simulink model "SPWMinverter3P_Final"  (Simulink 10.0)
settings: Solver=ode3  StartTime=0.0  StopTime=0.04  RelTol=1e-3  EnableMultiTasking=on
libraries: powerlib x16
settings Model: Creator=Administrator  LastModifiedBy=bhisma
settings SolverCC: PositivePriorityOrder=on
settings DataIOCC: LimitDataPoints=on  SignalLoggingSaveFormat=ModelDataLogs
settings OptimizationCC: ExpressionDepthLimit=2147483647
settings DebuggingCC: SolverPrmCheckMsg=warning  FcnCallInpInsideContextMsg=warning  StateNameClashWarn=warning
settings SFSimCC: SimParseCustomCode=off
settings GRTTargetCC: GeneratePreprocessorConditionals=Disable all
settings ConfigComp: CovExternalEMLEnable=off
settings SimscapeCC: SimscapeNormalizeSystem=off

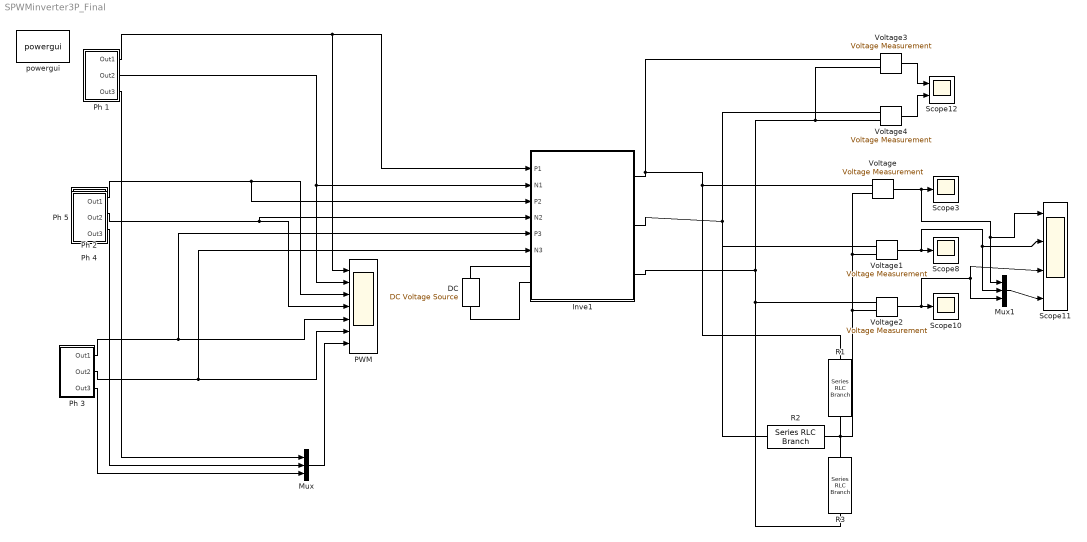
== system SPWMinverter3P_Final ==
  DC : powerlib/Electrical Sources/DC Voltage Source  SystemSampleTime=-1  Amplitude=10  Measurements=None
      settings: SourceProductName=Simscape Electrical
  Inve1 : Subsystem
  Mux : Mux  Inputs=3
  Mux1 : Mux  Inputs=3
  PWM : Scope  NumInputPorts=7
  Ph 1 : Subsystem  mask{SA=3, CA=3, Sf=50, Cf=5000}
      mask prompts: SA "Sine Amplitude"; CA "Carrier Amplitude"; Sf "Sine Frequency"; Cf "Carrier Frequency"
  Ph 2 : Subsystem  mask{SA=3, CA=3, Sf=50, Cf=5000}
      mask prompts: SA "Sine Amplitude"; CA "Carrier Amplitude"; Sf "Sine Frequency"; Cf "Carrier Frequency"
  Ph 3 : Subsystem  mask{SA=3, CA=3, Sf=50, Cf=5000}
      mask prompts: SA "Sine Amplitude"; CA "Carrier Amplitude"; Sf "Sine Frequency"; Cf "Carrier Frequency"
  Ph 4 : Subsystem  mask{SA=3, CA=3, Sf=50, Cf=5000}
      mask prompts: SA "Sine Amplitude"; CA "Carrier Amplitude"; Sf "Sine Frequency"; Cf "Carrier Frequency"
  Ph 5 : Subsystem  mask{SA=3, CA=3, Sf=50, Cf=5000}
      mask prompts: SA "Sine Amplitude"; CA "Carrier Amplitude"; Sf "Sine Frequency"; Cf "Carrier Frequency"
  R1 : powerlib/Elements/Series RLC Branch  PhysicalDomain=powersysdomain  SubClassName=unknown  LeftPortType=p1  RightPortType=p1  LConnTagsString=__new0  RConnTagsString=__new0  BranchType=R  Resistance=10  Inductance=1e-3  SetiL0=off  InitialCurrent=0  Capacitance=1e-6  Setx0=off  InitialVoltage=0  Measurements=None
      settings: SourceProductName=Simscape Electrical
  R2 : powerlib/Elements/Series RLC Branch  PhysicalDomain=powersysdomain  SubClassName=unknown  LeftPortType=p1  RightPortType=p1  LConnTagsString=__new0  RConnTagsString=__new0  BranchType=R  Resistance=10  Inductance=1e-3  SetiL0=off  InitialCurrent=0  Capacitance=1e-6  Setx0=off  InitialVoltage=0  Measurements=None
      settings: SourceProductName=Simscape Electrical
  R3 : powerlib/Elements/Series RLC Branch  PhysicalDomain=powersysdomain  SubClassName=unknown  LeftPortType=p1  RightPortType=p1  LConnTagsString=__new0  RConnTagsString=__new0  BranchType=R  Resistance=10  Inductance=1e-3  SetiL0=off  InitialCurrent=0  Capacitance=1e-6  Setx0=off  InitialVoltage=0  Measurements=None
      settings: SourceProductName=Simscape Electrical
  Scope10 : Scope
  Scope11 : Scope  NumInputPorts=4
  Scope12 : Scope  NumInputPorts=2
  Scope3 : Scope
  Scope8 : Scope
  Voltage{,1..4} (5 alike) : powerlib/Measurements/Voltage Measurement  SystemSampleTime=-1  PhasorSimulation=off  OutputType=Complex  PSBequivalent=0
      settings: SourceProductName=Simscape Electrical
  powergui : powerlib/powergui  Priority=1  SystemSampleTime=-1  SimulationMode=Continuous  SampleTime=50e-6  frequency=60  SPID=off  DisableSnubberDevices=off  DisableRonSwitches=off  DisableVfSwitches=off  SwTol=0  Interpol=off  frequencyindice=0  echomessages=off  HookPort=off  DisplayEquations=off  FunctionMessages=off  EnableUseOfTLC=off  x0status=blocks  RestoreLinks=warning  ResistiveCurrentMeasurement=off  Ylog=off  Xlog=on  ShowGrid=off  save=off  variable=ZData  ZoomFFT=off  StartTime=0.0  cycles=1  DisplayStyle=1  FreqAxis=off  MaxFrequency=1000  frequencyindicesteady=1  display=off  methode=off
      settings: SourceProductName=Simscape Electrical
  wires:
  Voltage/1 -> Scope11/1, Mux1/1, Scope3/1
  Mux/1 -> PWM/7
  Voltage1/1 -> Scope8/1, Scope11/2, Mux1/2
  Voltage2/1 -> Scope10/1, Scope11/3, Mux1/3
  Mux1/1 -> Scope11/4
  Voltage3/1 -> Scope12/1
  Voltage4/1 -> Scope12/2
  Ph 1/1(Out1) -> Inve1/1(P1), PWM/1
  Ph 1/2(Out2) -> Inve1/2(N1), PWM/2
  Ph 1/3(Out3) -> Mux/1
  Ph 2/1(Out1) -> Inve1/3(P2), PWM/3
  Ph 2/2(Out2) -> Inve1/4(N2), PWM/4
  Ph 2/3(Out3) -> Mux/2
  Ph 3/1(Out1) -> Inve1/5(P3), PWM/5
  Ph 3/2(Out2) -> Inve1/6(N3), PWM/6
  Ph 3/3(Out3) -> Mux/3
  connections:
  DC/RConn1 -- Inve1/LConn1
  Inve1/LConn2 -- DC/LConn1
  R1/RConn1 -- Voltage2/LConn2 -- Voltage1/LConn2 -- Voltage/LConn2 -- R3/RConn1 -- R2/LConn1
  R2/RConn1 -- Inve1/RConn2 -- Voltage4/LConn1 -- Voltage1/LConn1
  R3/LConn1 -- Voltage2/LConn1 -- Inve1/RConn3 -- Voltage4/LConn2 -- Voltage3/LConn2
  Inve1/RConn1 -- Voltage3/LConn1 -- R1/LConn1 -- Voltage/LConn1

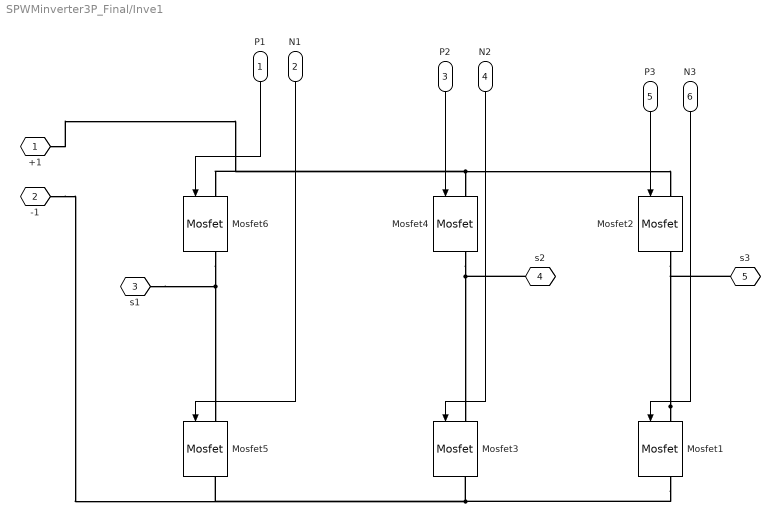
== system SPWMinverter3P_Final/Inve1 ==
  P1 : Inport
  N1 : Inport  Port=2
  P2 : Inport  Port=3
  N2 : Inport  Port=4
  P3 : Inport  Port=5
  N3 : Inport  Port=6
  Mosfet{1..6} (6 alike) : powerlib/Power Electronics/Mosfet  SystemSampleTime=-1  Ron=0.1  Lon=0  Rd=0.01  Vfd=0  IC=0  Rs=1e5  Cs=inf  Measurements=on
      settings: SourceProductName=Simscape Electrical
  +1 : PMIOPort  Tag=PMCPort  Side=Left
  -1 : PMIOPort  Tag=PMCPort  Port=2  Side=Left
  s1 : PMIOPort  Tag=PMCPort  Port=3  Side=Right
  s2 : PMIOPort  Tag=PMCPort  Port=4  Side=Right
  s3 : PMIOPort  Tag=PMCPort  Port=5  Side=Right
  wires:
  P1/1 -> Mosfet6/1
  N1/1 -> Mosfet5/1
  P2/1 -> Mosfet4/1
  N2/1 -> Mosfet3/1
  P3/1 -> Mosfet2/1
  N3/1 -> Mosfet1/1
  connections:
  Mosfet5/RConn1 -- -1/RConn1 -- Mosfet3/RConn1 -- Mosfet1/RConn1
  Mosfet6/LConn1 -- +1/RConn1 -- Mosfet4/LConn1 -- Mosfet2/LConn1
  Mosfet6/RConn1 -- Mosfet5/LConn1 -- s1/RConn1
  s2/RConn1 -- Mosfet4/RConn1 -- Mosfet3/LConn1
  Mosfet1/LConn1 -- s3/RConn1 -- Mosfet2/RConn1

== system SPWMinverter3P_Final/Ph 1 ==
  PWM1 : Subsystem  mask{Deg=0}
      mask prompts: Deg "Degree"
  Scope : Scope  NumInputPorts=3
  Scope1 : Scope  NumInputPorts=4
  Out1 : Outport
  Out2 : Outport  Port=2
  Out3 : Outport  Port=3
  wires:
  PWM1/6(Out6) -> Scope1/3
  PWM1/5(Out5) -> Scope1/2, Out2/1
  PWM1/4(Out4) -> Scope1/1, Out1/1
  PWM1/3(Out3) -> Scope/3
  PWM1/2(Out2) -> Scope/2
  PWM1/1(Out1) -> Scope/1
  PWM1/7(Out7) -> Scope1/4, Out3/1

== system SPWMinverter3P_Final/Ph 2 ==
  PWM 2 : Subsystem  mask{Deg=120}
      mask prompts: Deg "Degree"
  Scope2 : Scope  NumInputPorts=3
  Scope4 : Scope  NumInputPorts=4
  Out1 : Outport
  Out2 : Outport  Port=2
  Out3 : Outport  Port=3
  wires:
  PWM 2/6(Out6) -> Scope4/3
  PWM 2/5(Out5) -> Scope4/2, Out2/1
  PWM 2/4(Out4) -> Scope4/1, Out1/1
  PWM 2/3(Out3) -> Scope2/3
  PWM 2/2(Out2) -> Scope2/2
  PWM 2/1(Out1) -> Scope2/1
  PWM 2/7(Out7) -> Scope4/4, Out3/1

== system SPWMinverter3P_Final/Ph 3 ==
  PWM 3 : Subsystem  mask{Deg=240}
      mask prompts: Deg "Degree"
  Scope5 : Scope  NumInputPorts=3
  Scope6 : Scope  NumInputPorts=4
  Out1 : Outport
  Out2 : Outport  Port=2
  Out3 : Outport  Port=3
  wires:
  PWM 3/6(Out6) -> Scope6/3
  PWM 3/5(Out5) -> Scope6/2, Out2/1
  PWM 3/4(Out4) -> Scope6/1, Out1/1
  PWM 3/3(Out3) -> Scope5/3
  PWM 3/2(Out2) -> Scope5/2
  PWM 3/1(Out1) -> Scope5/1
  PWM 3/7(Out7) -> Scope6/4, Out3/1

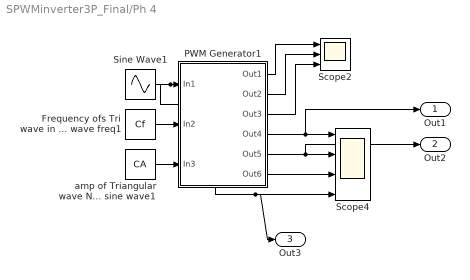
== system SPWMinverter3P_Final/Ph 4 ==
  Frequency ofs Tri wave in HZ note:It should < 2 times the sine wave freq1 : Constant  Value=Cf
  PWM Generator1 : Subsystem
  Scope2 : Scope  NumInputPorts=3
  Scope4 : Scope  NumInputPorts=4
  Sine Wave1 : Sin  Amplitude=SA  Frequency=2*pi*Sf  Phase=240*(pi/180)  SampleTime=0
  amp of Triangular wave Note:preferably the value of amp f sine wave1 : Constant  Value=CA
  Out1 : Outport
  Out2 : Outport  Port=2
  Out3 : Outport  Port=3
  wires:
  Sine Wave1/1 -> Out3/1, Scope4/4, PWM Generator1/1(In1)
  Frequency ofs Tri wave in HZ note:It should < 2 times the sine wave freq1/1 -> PWM Generator1/2(In2)
  amp of Triangular wave Note:preferably the value of amp f sine wave1/1 -> PWM Generator1/3(In3)
  PWM Generator1/1(Out1) -> Scope2/1
  PWM Generator1/2(Out2) -> Scope2/2
  PWM Generator1/3(Out3) -> Scope2/3
  PWM Generator1/4(Out4) -> Out1/1, Scope4/1
  PWM Generator1/5(Out5) -> Out2/1, Scope4/2
  PWM Generator1/6(Out6) -> Scope4/3

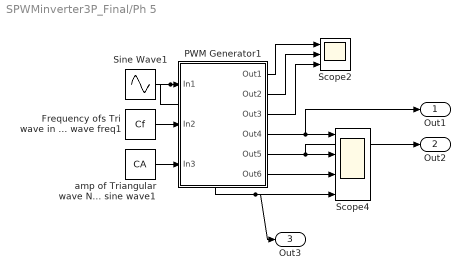
== system SPWMinverter3P_Final/Ph 5 ==
  Frequency ofs Tri wave in HZ note:It should < 2 times the sine wave freq1 : Constant  Value=Cf
  PWM Generator1 : Subsystem
  Scope2 : Scope  NumInputPorts=3
  Scope4 : Scope  NumInputPorts=4
  Sine Wave1 : Sin  Amplitude=SA  Frequency=2*pi*Sf  Phase=120*(pi/180)  SampleTime=0
  amp of Triangular wave Note:preferably the value of amp f sine wave1 : Constant  Value=CA
  Out1 : Outport
  Out2 : Outport  Port=2
  Out3 : Outport  Port=3
  wires:
  Sine Wave1/1 -> Out3/1, Scope4/4, PWM Generator1/1(In1)
  Frequency ofs Tri wave in HZ note:It should < 2 times the sine wave freq1/1 -> PWM Generator1/2(In2)
  amp of Triangular wave Note:preferably the value of amp f sine wave1/1 -> PWM Generator1/3(In3)
  PWM Generator1/1(Out1) -> Scope2/1
  PWM Generator1/2(Out2) -> Scope2/2
  PWM Generator1/3(Out3) -> Scope2/3
  PWM Generator1/4(Out4) -> Out1/1, Scope4/1
  PWM Generator1/5(Out5) -> Out2/1, Scope4/2
  PWM Generator1/6(Out6) -> Scope4/3

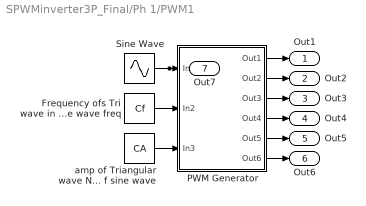
== system SPWMinverter3P_Final/Ph 1/PWM1 ==
  Frequency ofs Tri wave in HZ note:It should < 2 times the sine wave freq : Constant  Value=Cf
  PWM Generator : Subsystem
  Sine Wave : Sin  Amplitude=SA  Frequency=2*pi*Sf  Phase=Deg  SampleTime=0
  amp of Triangular wave Note:preferably the value of amp f sine wave : Constant  Value=CA
  Out1 : Outport
  Out2 : Outport  Port=2
  Out3 : Outport  Port=3
  Out4 : Outport  Port=4
  Out5 : Outport  Port=5
  Out6 : Outport  Port=6
  Out7 : Outport  Port=7
  wires:
  amp of Triangular wave Note:preferably the value of amp f sine wave/1 -> PWM Generator/3(In3)
  Frequency ofs Tri wave in HZ note:It should < 2 times the sine wave freq/1 -> PWM Generator/2(In2)
  Sine Wave/1 -> PWM Generator/1(In1), Out7/1
  PWM Generator/1(Out1) -> Out1/1
  PWM Generator/2(Out2) -> Out2/1
  PWM Generator/3(Out3) -> Out3/1
  PWM Generator/4(Out4) -> Out4/1
  PWM Generator/5(Out5) -> Out5/1
  PWM Generator/6(Out6) -> Out6/1

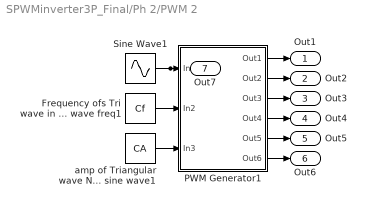
== system SPWMinverter3P_Final/Ph 2/PWM 2 ==
  Frequency ofs Tri wave in HZ note:It should < 2 times the sine wave freq1 : Constant  Value=Cf
  PWM Generator1 : Subsystem
  Sine Wave1 : Sin  Amplitude=SA  Frequency=2*pi*Sf  Phase=Deg*(pi/180)  SampleTime=0
  amp of Triangular wave Note:preferably the value of amp f sine wave1 : Constant  Value=CA
  Out1 : Outport
  Out2 : Outport  Port=2
  Out3 : Outport  Port=3
  Out4 : Outport  Port=4
  Out5 : Outport  Port=5
  Out6 : Outport  Port=6
  Out7 : Outport  Port=7
  wires:
  amp of Triangular wave Note:preferably the value of amp f sine wave1/1 -> PWM Generator1/3(In3)
  Frequency ofs Tri wave in HZ note:It should < 2 times the sine wave freq1/1 -> PWM Generator1/2(In2)
  Sine Wave1/1 -> PWM Generator1/1(In1), Out7/1
  PWM Generator1/1(Out1) -> Out1/1
  PWM Generator1/2(Out2) -> Out2/1
  PWM Generator1/3(Out3) -> Out3/1
  PWM Generator1/4(Out4) -> Out4/1
  PWM Generator1/5(Out5) -> Out5/1
  PWM Generator1/6(Out6) -> Out6/1

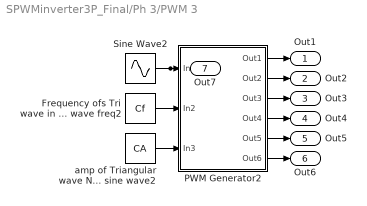
== system SPWMinverter3P_Final/Ph 3/PWM 3 ==
  Frequency ofs Tri wave in HZ note:It should < 2 times the sine wave freq2 : Constant  Value=Cf
  PWM Generator2 : Subsystem
  Sine Wave2 : Sin  Amplitude=SA  Frequency=2*pi*Sf  Phase=Deg*(pi/180)  SampleTime=0
  amp of Triangular wave Note:preferably the value of amp f sine wave2 : Constant  Value=CA
  Out1 : Outport
  Out2 : Outport  Port=2
  Out3 : Outport  Port=3
  Out4 : Outport  Port=4
  Out5 : Outport  Port=5
  Out6 : Outport  Port=6
  Out7 : Outport  Port=7
  wires:
  amp of Triangular wave Note:preferably the value of amp f sine wave2/1 -> PWM Generator2/3(In3)
  Frequency ofs Tri wave in HZ note:It should < 2 times the sine wave freq2/1 -> PWM Generator2/2(In2)
  Sine Wave2/1 -> PWM Generator2/1(In1), Out7/1
  PWM Generator2/1(Out1) -> Out1/1
  PWM Generator2/2(Out2) -> Out2/1
  PWM Generator2/3(Out3) -> Out3/1
  PWM Generator2/4(Out4) -> Out4/1
  PWM Generator2/5(Out5) -> Out5/1
  PWM Generator2/6(Out6) -> Out6/1

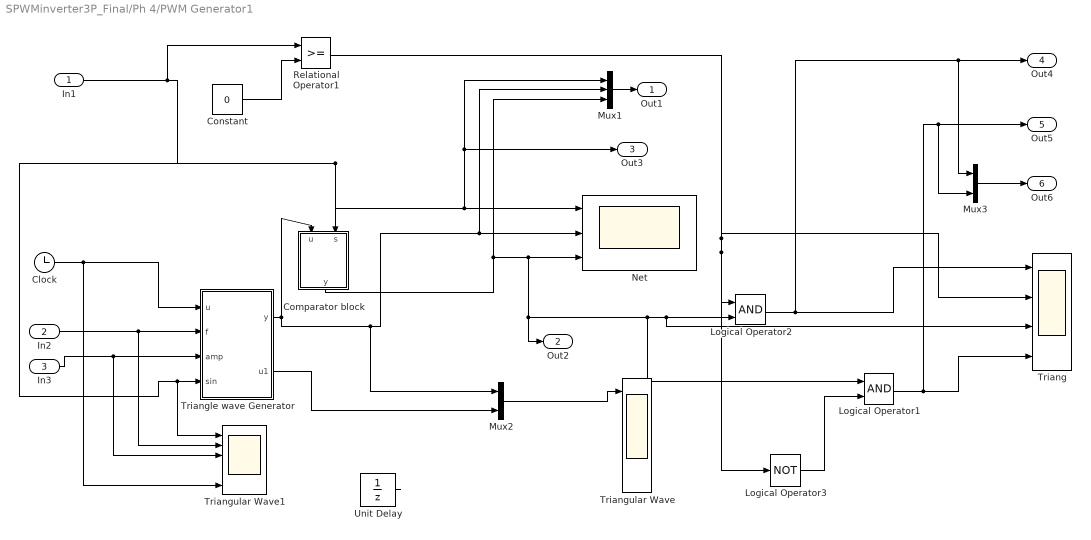
== system SPWMinverter3P_Final/Ph 4/PWM Generator1 ==
  In1 : Inport
  In2 : Inport  Port=2
  In3 : Inport  Port=3
  Clock : Clock
  Comparator block : MATLAB Function  TreatAsAtomicUnit=on
  Constant : Constant  Value=0
  Logical Operator1 : Logic  AllPortsSameDT=off  OutDataTypeStr=boolean
  Logical Operator2 : Logic  AllPortsSameDT=off  OutDataTypeStr=boolean
  Logical Operator3 : Logic  Operator=NOT  AllPortsSameDT=off  OutDataTypeStr=boolean
  Mux1 : Mux  Inputs=3
  Mux2 : Mux  Inputs=2
  Mux3 : Mux  Inputs=2
  Net : Scope  NumInputPorts=3
  Relational Operator1 : RelationalOperator  RndMeth=Nearest  InputSameDT=on
  Triang : Scope  NumInputPorts=4
  Triangle wave Generator : MATLAB Function  TreatAsAtomicUnit=on
  Triangular Wave : Scope  NumInputPorts=4
  Triangular Wave1 : Scope  NumInputPorts=6
  Unit Delay : UnitDelay  SampleTime=.01/10000
  Out1 : Outport
  Out2 : Outport  Port=2
  Out3 : Outport  Port=3
  Out4 : Outport  Port=4
  Out5 : Outport  Port=5
  Out6 : Outport  Port=6
  wires:
  Mux3/1 -> Out6/1
  Logical Operator1/1 -> Mux3/2, Out5/1, Triang/4
  Logical Operator3/1 -> Logical Operator1/2
  Logical Operator2/1 -> Mux3/1, Out4/1, Triang/1
  Relational Operator1/1 -> Logical Operator3/1, Logical Operator2/1, Triang/2
  Constant/1 -> Relational Operator1/2
  In3/1 -> Triangular Wave1/3, Triangle wave Generator/3(amp)
  In2/1 -> Triangular Wave1/2, Triangle wave Generator/2(f)
  Mux1/1 -> Out1/1
  Mux2/1 -> Triangular Wave/1
  Triangle wave Generator/2(u1) -> Mux2/2
  Comparator block/1(y) -> Logical Operator1/1, Triang/3, Logical Operator2/2, Out2/1, Net/3, Mux1/3
  In1/1 -> Relational Operator1/1, Triangular Wave1/1, Triangle wave Generator/4(sin), Comparator block/2(s), Net/1, Out3/1, Mux1/1
  Unit Delay/1 -> Unit Delay/1
  Triangle wave Generator/1(y) -> Mux2/1, Net/2, Mux1/2, Comparator block/1(u)
  Clock/1 -> Triangular Wave1/6, Triangle wave Generator/1(u)

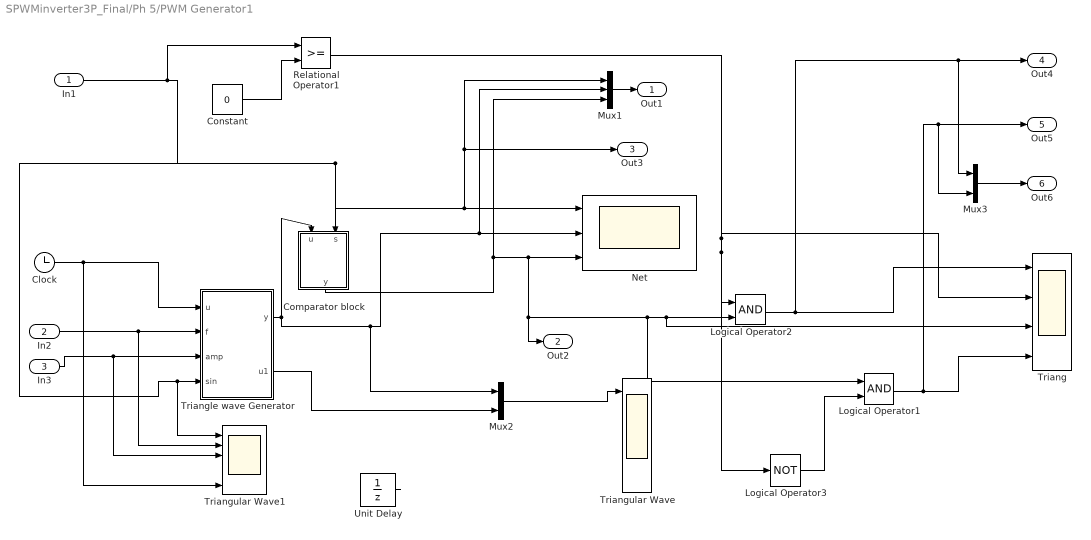
== system SPWMinverter3P_Final/Ph 5/PWM Generator1 ==
  In1 : Inport
  In2 : Inport  Port=2
  In3 : Inport  Port=3
  Clock : Clock
  Comparator block : MATLAB Function  TreatAsAtomicUnit=on
  Constant : Constant  Value=0
  Logical Operator1 : Logic  AllPortsSameDT=off  OutDataTypeStr=boolean
  Logical Operator2 : Logic  AllPortsSameDT=off  OutDataTypeStr=boolean
  Logical Operator3 : Logic  Operator=NOT  AllPortsSameDT=off  OutDataTypeStr=boolean
  Mux1 : Mux  Inputs=3
  Mux2 : Mux  Inputs=2
  Mux3 : Mux  Inputs=2
  Net : Scope  NumInputPorts=3
  Relational Operator1 : RelationalOperator  RndMeth=Nearest  InputSameDT=on
  Triang : Scope  NumInputPorts=4
  Triangle wave Generator : MATLAB Function  TreatAsAtomicUnit=on
  Triangular Wave : Scope  NumInputPorts=4
  Triangular Wave1 : Scope  NumInputPorts=6
  Unit Delay : UnitDelay  SampleTime=.01/10000
  Out1 : Outport
  Out2 : Outport  Port=2
  Out3 : Outport  Port=3
  Out4 : Outport  Port=4
  Out5 : Outport  Port=5
  Out6 : Outport  Port=6
  wires:
  Mux3/1 -> Out6/1
  Logical Operator1/1 -> Mux3/2, Out5/1, Triang/4
  Logical Operator3/1 -> Logical Operator1/2
  Logical Operator2/1 -> Mux3/1, Out4/1, Triang/1
  Relational Operator1/1 -> Logical Operator3/1, Logical Operator2/1, Triang/2
  Constant/1 -> Relational Operator1/2
  In3/1 -> Triangular Wave1/3, Triangle wave Generator/3(amp)
  In2/1 -> Triangular Wave1/2, Triangle wave Generator/2(f)
  Mux1/1 -> Out1/1
  Mux2/1 -> Triangular Wave/1
  Triangle wave Generator/2(u1) -> Mux2/2
  Comparator block/1(y) -> Logical Operator1/1, Triang/3, Logical Operator2/2, Out2/1, Net/3, Mux1/3
  In1/1 -> Relational Operator1/1, Triangular Wave1/1, Triangle wave Generator/4(sin), Comparator block/2(s), Net/1, Out3/1, Mux1/1
  Unit Delay/1 -> Unit Delay/1
  Triangle wave Generator/1(y) -> Mux2/1, Net/2, Mux1/2, Comparator block/1(u)
  Clock/1 -> Triangular Wave1/6, Triangle wave Generator/1(u)

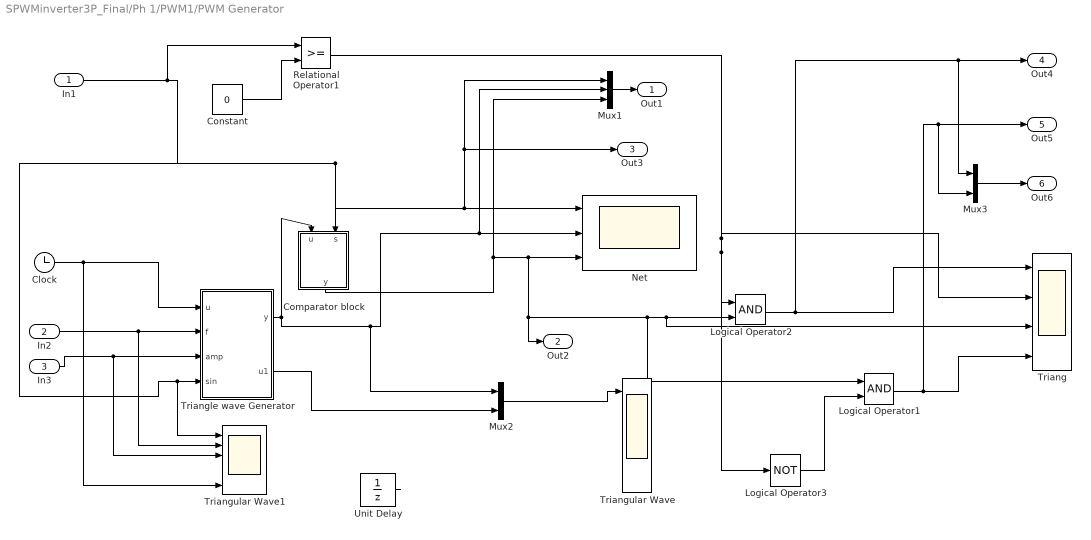
== system SPWMinverter3P_Final/Ph 1/PWM1/PWM Generator ==
  In1 : Inport
  In2 : Inport  Port=2
  In3 : Inport  Port=3
  Clock : Clock
  Comparator block : MATLAB Function  TreatAsAtomicUnit=on
  Constant : Constant  Value=0
  Logical Operator1 : Logic  AllPortsSameDT=off  OutDataTypeStr=boolean
  Logical Operator2 : Logic  AllPortsSameDT=off  OutDataTypeStr=boolean
  Logical Operator3 : Logic  Operator=NOT  AllPortsSameDT=off  OutDataTypeStr=boolean
  Mux1 : Mux  Inputs=3
  Mux2 : Mux  Inputs=2
  Mux3 : Mux  Inputs=2
  Net : Scope  NumInputPorts=3
  Relational Operator1 : RelationalOperator  RndMeth=Nearest  InputSameDT=on
  Triang : Scope  NumInputPorts=4
  Triangle wave Generator : MATLAB Function  TreatAsAtomicUnit=on
  Triangular Wave : Scope  NumInputPorts=4
  Triangular Wave1 : Scope  NumInputPorts=6
  Unit Delay : UnitDelay  SampleTime=.01/10000
  Out1 : Outport
  Out2 : Outport  Port=2
  Out3 : Outport  Port=3
  Out4 : Outport  Port=4
  Out5 : Outport  Port=5
  Out6 : Outport  Port=6
  wires:
  Clock/1 -> Triangle wave Generator/1(u), Triangular Wave1/6
  Triangle wave Generator/1(y) -> Comparator block/1(u), Mux1/2, Net/2, Mux2/1
  Unit Delay/1 -> Unit Delay/1
  In1/1 -> Mux1/1, Out3/1, Net/1, Comparator block/2(s), Triangle wave Generator/4(sin), Triangular Wave1/1, Relational Operator1/1
  Comparator block/1(y) -> Mux1/3, Net/3, Out2/1, Logical Operator2/2, Triang/3, Logical Operator1/1
  Triangle wave Generator/2(u1) -> Mux2/2
  Mux2/1 -> Triangular Wave/1
  Mux1/1 -> Out1/1
  In2/1 -> Triangle wave Generator/2(f), Triangular Wave1/2
  In3/1 -> Triangle wave Generator/3(amp), Triangular Wave1/3
  Constant/1 -> Relational Operator1/2
  Relational Operator1/1 -> Triang/2, Logical Operator2/1, Logical Operator3/1
  Logical Operator2/1 -> Triang/1, Out4/1, Mux3/1
  Logical Operator3/1 -> Logical Operator1/2
  Logical Operator1/1 -> Triang/4, Out5/1, Mux3/2
  Mux3/1 -> Out6/1

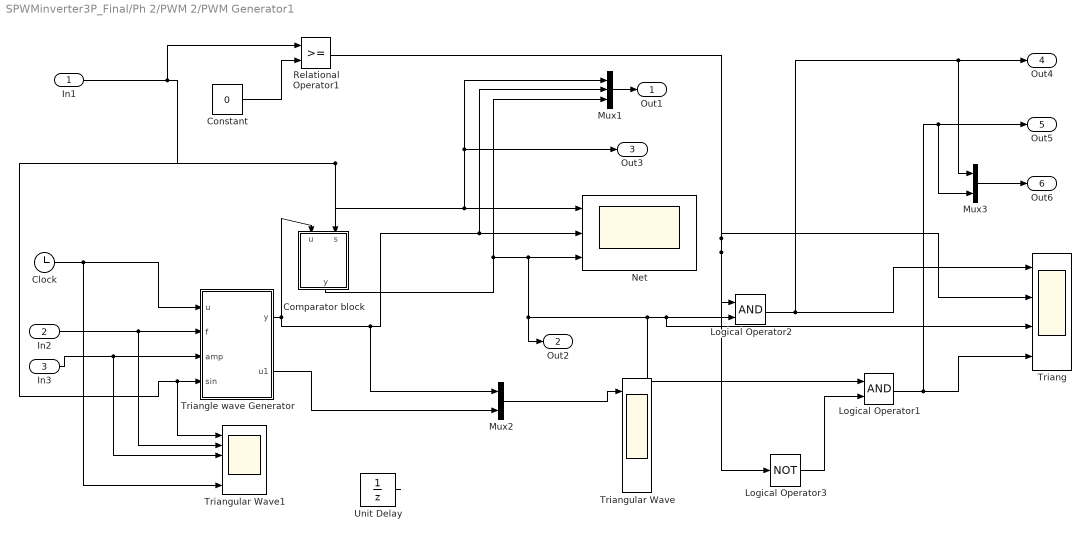
== system SPWMinverter3P_Final/Ph 2/PWM 2/PWM Generator1 ==
  In1 : Inport
  In2 : Inport  Port=2
  In3 : Inport  Port=3
  Clock : Clock
  Comparator block : MATLAB Function  TreatAsAtomicUnit=on
  Constant : Constant  Value=0
  Logical Operator1 : Logic  AllPortsSameDT=off  OutDataTypeStr=boolean
  Logical Operator2 : Logic  AllPortsSameDT=off  OutDataTypeStr=boolean
  Logical Operator3 : Logic  Operator=NOT  AllPortsSameDT=off  OutDataTypeStr=boolean
  Mux1 : Mux  Inputs=3
  Mux2 : Mux  Inputs=2
  Mux3 : Mux  Inputs=2
  Net : Scope  NumInputPorts=3
  Relational Operator1 : RelationalOperator  RndMeth=Nearest  InputSameDT=on
  Triang : Scope  NumInputPorts=4
  Triangle wave Generator : MATLAB Function  TreatAsAtomicUnit=on
  Triangular Wave : Scope  NumInputPorts=4
  Triangular Wave1 : Scope  NumInputPorts=6
  Unit Delay : UnitDelay  SampleTime=.01/10000
  Out1 : Outport
  Out2 : Outport  Port=2
  Out3 : Outport  Port=3
  Out4 : Outport  Port=4
  Out5 : Outport  Port=5
  Out6 : Outport  Port=6
  wires:
  Clock/1 -> Triangle wave Generator/1(u), Triangular Wave1/6
  Triangle wave Generator/1(y) -> Comparator block/1(u), Mux1/2, Net/2, Mux2/1
  Unit Delay/1 -> Unit Delay/1
  In1/1 -> Mux1/1, Out3/1, Net/1, Comparator block/2(s), Triangle wave Generator/4(sin), Triangular Wave1/1, Relational Operator1/1
  Comparator block/1(y) -> Mux1/3, Net/3, Out2/1, Logical Operator2/2, Triang/3, Logical Operator1/1
  Triangle wave Generator/2(u1) -> Mux2/2
  Mux2/1 -> Triangular Wave/1
  Mux1/1 -> Out1/1
  In2/1 -> Triangle wave Generator/2(f), Triangular Wave1/2
  In3/1 -> Triangle wave Generator/3(amp), Triangular Wave1/3
  Constant/1 -> Relational Operator1/2
  Relational Operator1/1 -> Triang/2, Logical Operator2/1, Logical Operator3/1
  Logical Operator2/1 -> Triang/1, Out4/1, Mux3/1
  Logical Operator3/1 -> Logical Operator1/2
  Logical Operator1/1 -> Triang/4, Out5/1, Mux3/2
  Mux3/1 -> Out6/1

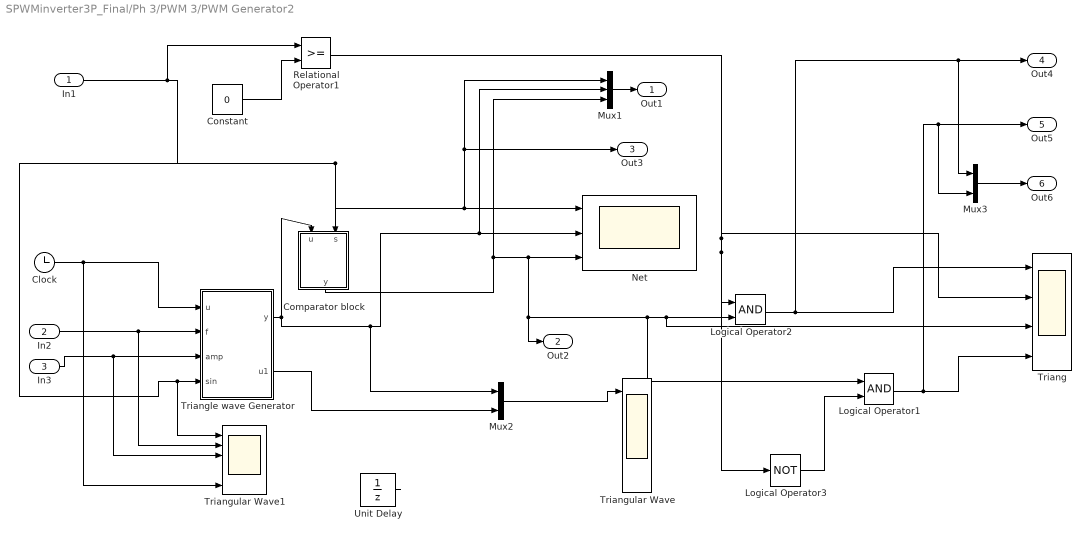
== system SPWMinverter3P_Final/Ph 3/PWM 3/PWM Generator2 ==
  In1 : Inport
  In2 : Inport  Port=2
  In3 : Inport  Port=3
  Clock : Clock
  Comparator block : MATLAB Function  TreatAsAtomicUnit=on
  Constant : Constant  Value=0
  Logical Operator1 : Logic  AllPortsSameDT=off  OutDataTypeStr=boolean
  Logical Operator2 : Logic  AllPortsSameDT=off  OutDataTypeStr=boolean
  Logical Operator3 : Logic  Operator=NOT  AllPortsSameDT=off  OutDataTypeStr=boolean
  Mux1 : Mux  Inputs=3
  Mux2 : Mux  Inputs=2
  Mux3 : Mux  Inputs=2
  Net : Scope  NumInputPorts=3
  Relational Operator1 : RelationalOperator  RndMeth=Nearest  InputSameDT=on
  Triang : Scope  NumInputPorts=4
  Triangle wave Generator : MATLAB Function  TreatAsAtomicUnit=on
  Triangular Wave : Scope  NumInputPorts=4
  Triangular Wave1 : Scope  NumInputPorts=6
  Unit Delay : UnitDelay  SampleTime=.01/10000
  Out1 : Outport
  Out2 : Outport  Port=2
  Out3 : Outport  Port=3
  Out4 : Outport  Port=4
  Out5 : Outport  Port=5
  Out6 : Outport  Port=6
  wires:
  Clock/1 -> Triangle wave Generator/1(u), Triangular Wave1/6
  Triangle wave Generator/1(y) -> Comparator block/1(u), Mux1/2, Net/2, Mux2/1
  Unit Delay/1 -> Unit Delay/1
  In1/1 -> Mux1/1, Out3/1, Net/1, Comparator block/2(s), Triangle wave Generator/4(sin), Triangular Wave1/1, Relational Operator1/1
  Comparator block/1(y) -> Mux1/3, Net/3, Out2/1, Logical Operator2/2, Triang/3, Logical Operator1/1
  Triangle wave Generator/2(u1) -> Mux2/2
  Mux2/1 -> Triangular Wave/1
  Mux1/1 -> Out1/1
  In2/1 -> Triangle wave Generator/2(f), Triangular Wave1/2
  In3/1 -> Triangle wave Generator/3(amp), Triangular Wave1/3
  Constant/1 -> Relational Operator1/2
  Relational Operator1/1 -> Triang/2, Logical Operator2/1, Logical Operator3/1
  Logical Operator2/1 -> Triang/1, Out4/1, Mux3/1
  Logical Operator3/1 -> Logical Operator1/2
  Logical Operator1/1 -> Triang/4, Out5/1, Mux3/2
  Mux3/1 -> Out6/1

== matlab function Ph 1/PWM1/PWM Generator/Comparator block ==
  data: u input double; y output double; s input double
function y  = fcn(u,s)
%#eml
if(s>=0)
if(s>=u)
    y = 5;
 else
    y=0;
end
else if(s<=u)
    y=5;
 else
    y=0;
    end
end

== matlab function Ph 1/PWM1/PWM Generator/Triangle wave Generator ==
  data: u input double; y output double; f input double; amp input double; sin input double; u1 output double
function [y,u1]= fcn(u,f,amp,sin)
%#eml

%a=amp*1000*2;%wrong method 
%if amplitude is 'a' means peak to peak is 'a'. but if sine wave amp is 'a' peak to peak is '2a'
%hence multiplying the value of 'a' (for triangle wave)with 2.hence we can compare with sine wave
%the above statement is pure "wrong" undestanding. 
t=1/f;%0.04-time period
t1=t/2;%0.02

a=amp/t1;%finding the multiplication factor from the amp and time period
%for eg. for freq 5000,t1=.0001 
%but for freq 500 , t1=.001 
%so the amplitude of triangular wave will vary depending upon the freq if we dont use this formula.
%but still it cant generate a triangular wave for freq value of less than sine wave freq.(we are taking sine wave as ref 
%to generate positive and negative half cycle of triangular wave

if(u>t)
    u=rem(u,t) %to make the clock cycle to zero @ time t(repeating sequence)
end

u1=u*1000;%to plot the u values
%1000 is to magnify

if(u>=1.99&&u<=2.01) %error correction - to make 0 @ time 2
    y=0;
elseif(u<t1)
    if(sin>=0)%checking whether the sine wave is positive or not.If sine is +ve Triangluar is +ve
        %if sine is negative triangula is negative
    y = u*a;%increasing
    else
    y = -(u*a); 
    end

else
    if(sin>=0)
    y=a*(abs((rem(u,t1)-t1)));%decreasing
    else
    y=-a*((abs((rem(u,t1)-t1)))); 
    end
    
end

== matlab function Ph 2/PWM 2/PWM Generator1/Comparator block ==
  data: u input double; y output double; s input double
function y  = fcn(u,s)
%#eml
if(s>=0)
if(s>=u)
    y = 5;
 else
    y=0;
end
else if(s<=u)
    y=5;
 else
    y=0;
    end
end

== matlab function Ph 2/PWM 2/PWM Generator1/Triangle wave Generator ==
  data: u input double; y output double; f input double; amp input double; sin input double; u1 output double
function [y,u1]= fcn(u,f,amp,sin)
%#eml

%a=amp*1000*2;%wrong method 
%if amplitude is 'a' means peak to peak is 'a'. but if sine wave amp is 'a' peak to peak is '2a'
%hence multiplying the value of 'a' (for triangle wave)with 2.hence we can compare with sine wave
%the above statement is pure "wrong" undestanding. 
t=1/f;%0.04-time period
t1=t/2;%0.02

a=amp/t1;%finding the multiplication factor from the amp and time period
%for eg. for freq 5000,t1=.0001 
%but for freq 500 , t1=.001 
%so the amplitude of triangular wave will vary depending upon the freq if we dont use this formula.
%but still it cant generate a triangular wave for freq value of less than sine wave freq.(we are taking sine wave as ref 
%to generate positive and negative half cycle of triangular wave

if(u>t)
    u=rem(u,t) %to make the clock cycle to zero @ time t(repeating sequence)
end

u1=u*1000;%to plot the u values
%1000 is to magnify

if(u>=1.99&&u<=2.01) %error correction - to make 0 @ time 2
    y=0;
elseif(u<t1)
    if(sin>=0)%checking whether the sine wave is positive or not.If sine is +ve Triangluar is +ve
        %if sine is negative triangula is negative
    y = u*a;%increasing
    else
    y = -(u*a); 
    end

else
    if(sin>=0)
    y=a*(abs((rem(u,t1)-t1)));%decreasing
    else
    y=-a*((abs((rem(u,t1)-t1)))); 
    end
    
end

== matlab function Ph 3/PWM 3/PWM Generator2/Comparator block ==
  data: u input double; y output double; s input double
function y  = fcn(u,s)
%#eml
if(s>=0)
if(s>=u)
    y = 5;
 else
    y=0;
end
else if(s<=u)
    y=5;
 else
    y=0;
    end
end

== matlab function Ph 3/PWM 3/PWM Generator2/Triangle wave Generator ==
  data: u input double; y output double; f input double; amp input double; sin input double; u1 output double
function [y,u1]= fcn(u,f,amp,sin)
%#eml

%a=amp*1000*2;%wrong method 
%if amplitude is 'a' means peak to peak is 'a'. but if sine wave amp is 'a' peak to peak is '2a'
%hence multiplying the value of 'a' (for triangle wave)with 2.hence we can compare with sine wave
%the above statement is pure "wrong" undestanding. 
t=1/f;%0.04-time period
t1=t/2;%0.02

a=amp/t1;%finding the multiplication factor from the amp and time period
%for eg. for freq 5000,t1=.0001 
%but for freq 500 , t1=.001 
%so the amplitude of triangular wave will vary depending upon the freq if we dont use this formula.
%but still it cant generate a triangular wave for freq value of less than sine wave freq.(we are taking sine wave as ref 
%to generate positive and negative half cycle of triangular wave

if(u>t)
    u=rem(u,t) %to make the clock cycle to zero @ time t(repeating sequence)
end

u1=u*1000;%to plot the u values
%1000 is to magnify

if(u>=1.99&&u<=2.01) %error correction - to make 0 @ time 2
    y=0;
elseif(u<t1)
    if(sin>=0)%checking whether the sine wave is positive or not.If sine is +ve Triangluar is +ve
        %if sine is negative triangula is negative
    y = u*a;%increasing
    else
    y = -(u*a); 
    end

else
    if(sin>=0)
    y=a*(abs((rem(u,t1)-t1)));%decreasing
    else
    y=-a*((abs((rem(u,t1)-t1)))); 
    end
    
end

== matlab function Ph 4/PWM Generator1/Comparator block ==
  data: u input double; y output double; s input double
function y  = fcn(u,s)
%#eml
if(s>=0)
if(s>=u)
    y = 5;
 else
    y=0;
end
else if(s<=u)
    y=5;
 else
    y=0;
    end
end

== matlab function Ph 4/PWM Generator1/Triangle wave Generator ==
  data: u input double; y output double; f input double; amp input double; sin input double; u1 output double
function [y,u1]= fcn(u,f,amp,sin)
%#eml

%a=amp*1000*2;%wrong method 
%if amplitude is 'a' means peak to peak is 'a'. but if sine wave amp is 'a' peak to peak is '2a'
%hence multiplying the value of 'a' (for triangle wave)with 2.hence we can compare with sine wave
%the above statement is pure "wrong" undestanding. 
t=1/f;%0.04-time period
t1=t/2;%0.02

a=amp/t1;%finding the multiplication factor from the amp and time period
%for eg. for freq 5000,t1=.0001 
%but for freq 500 , t1=.001 
%so the amplitude of triangular wave will vary depending upon the freq if we dont use this formula.
%but still it cant generate a triangular wave for freq value of less than sine wave freq.(we are taking sine wave as ref 
%to generate positive and negative half cycle of triangular wave

if(u>t)
    u=rem(u,t) %to make the clock cycle to zero @ time t(repeating sequence)
end

u1=u*1000;%to plot the u values
%1000 is to magnify

if(u>=1.99&&u<=2.01) %error correction - to make 0 @ time 2
    y=0;
elseif(u<t1)
    if(sin>=0)%checking whether the sine wave is positive or not.If sine is +ve Triangluar is +ve
        %if sine is negative triangula is negative
    y = u*a;%increasing
    else
    y = -(u*a); 
    end

else
    if(sin>=0)
    y=a*(abs((rem(u,t1)-t1)));%decreasing
    else
    y=-a*((abs((rem(u,t1)-t1)))); 
    end
    
end

== matlab function Ph 5/PWM Generator1/Comparator block ==
  data: u input double; y output double; s input double
function y  = fcn(u,s)
%#eml
if(s>=0)
if(s>=u)
    y = 5;
 else
    y=0;
end
else if(s<=u)
    y=5;
 else
    y=0;
    end
end

== matlab function Ph 5/PWM Generator1/Triangle wave Generator ==
  data: u input double; y output double; f input double; amp input double; sin input double; u1 output double
function [y,u1]= fcn(u,f,amp,sin)
%#eml

%a=amp*1000*2;%wrong method 
%if amplitude is 'a' means peak to peak is 'a'. but if sine wave amp is 'a' peak to peak is '2a'
%hence multiplying the value of 'a' (for triangle wave)with 2.hence we can compare with sine wave
%the above statement is pure "wrong" undestanding. 
t=1/f;%0.04-time period
t1=t/2;%0.02

a=amp/t1;%finding the multiplication factor from the amp and time period
%for eg. for freq 5000,t1=.0001 
%but for freq 500 , t1=.001 
%so the amplitude of triangular wave will vary depending upon the freq if we dont use this formula.
%but still it cant generate a triangular wave for freq value of less than sine wave freq.(we are taking sine wave as ref 
%to generate positive and negative half cycle of triangular wave

if(u>t)
    u=rem(u,t) %to make the clock cycle to zero @ time t(repeating sequence)
end

u1=u*1000;%to plot the u values
%1000 is to magnify

if(u>=1.99&&u<=2.01) %error correction - to make 0 @ time 2
    y=0;
elseif(u<t1)
    if(sin>=0)%checking whether the sine wave is positive or not.If sine is +ve Triangluar is +ve
        %if sine is negative triangula is negative
    y = u*a;%increasing
    else
    y = -(u*a); 
    end

else
    if(sin>=0)
    y=a*(abs((rem(u,t1)-t1)));%decreasing
    else
    y=-a*((abs((rem(u,t1)-t1)))); 
    end
    
end
